simulink model "component_planner_adaptive_MPC"  (R2025a)
settings: Solver=FixedStepAuto  StartTime=0.0  StopTime=100  FixedStep=0.01  RelTol=1e-3  EnableMultiTasking=on
undefined symbols (not defined in the file): ego_target_velocity, MPC_prediction_horizon, tgt_traj_accel, tgt_traj_angle, tgt_traj_cte, tgt_traj_curv, tgt_traj_pos_x, tgt_traj_pos_y, tgt_traj_time, tgt_traj_velo, traj_valid_points
libraries: mpclib x1
settings Model: PauseTimes=61  NumberOfSteps=100  Creator=Z145442  LastModifiedBy=MarikL
settings SolverCC: AlgebraicLoopSolver=TrustRegion  PositivePriorityOrder=on  AutoInsertRateTranBlk=on
settings DataIOCC: SaveOutput=off  DSMLogging=off  SaveTime=off
settings OptimizationCC: EnhancedBackFolding=on  PassReuseOutputArgsAs=Individual arguments  ZeroExternalMemoryAtStartup=off  ZeroInternalMemoryAtStartup=off  MaxStackSize=2048  OptimizeBlockOrder=speed  DifferentSizesBufferReuse=on  OptimizationCustomize=off  EfficientTunableParamExpr=on
settings DebuggingCC: SignalInfNanChecking=error  MergeDetectMultiDrivingBlocksExec=none  ParameterOverflowMsg=none  ParameterTunabilityLossMsg=error  UnconnectedInputMsg=warning  UnconnectedOutputMsg=warning  UnconnectedLineMsg=warning  UniqueDataStoreMsg=warning  SFNoUnconditionalDefaultTransitionDiag=warning  ArithmeticOperatorsInVariantConditions=warning
settings HardwareCC: ProdBitPerPointer=32.0  ProdBitPerSizeT=32.0  ProdBitPerPtrDiffT=32.0  ProdLargestAtomicInteger=Long  ProdWordSize=32.0  ProdLongLongMode=on  ProdHWDeviceType=Infineon->TriCore
settings ModelReferenceCC: EnableRefExpFcnMdlSchedulingChecks=on  ModelReferenceNumInstancesAllowed=Single
settings SFSimCC: SimUseLocalCustomCode=off  MATLABDynamicMemAlloc=off  CustomCodeUndefinedFunction=UseInterfaceOnly
settings RTWCC: SystemTargetFile=ert.tlc  HardwareBoard=Infineon AURIX TC4x - TriBoards  GenCodeOnly=on  TemplateMakefile=ert_default_tmf  RTWUseLocalCustomCode=off  Toolchain=TASKING SmartCode for TriCore  GPUComputeCapability=3.5  Description=Embedded Coder
settings CodeAppCC: ForceParamTrailComments=on  IgnoreCustomStorageClasses=off  MaxIdLength=256.0  OperatorAnnotations=on  SimulinkDataObjDesc=on  SFDataObjDesc=on  InsertBlockDesc=on
settings ERTTargetCC: ExtModeTransport=0.0  ExtModeStaticAlloc=off  ExtModeMexFile=ext_comm  ExtModeIntrfLevel=Level1  InlinedParameterPlacement=Hierarchical  DynamicArrayContainerType=coder::array  SubcomponentCodeInterfacePackaging=Nonreusable function  SupportVariableSizeSignals=on

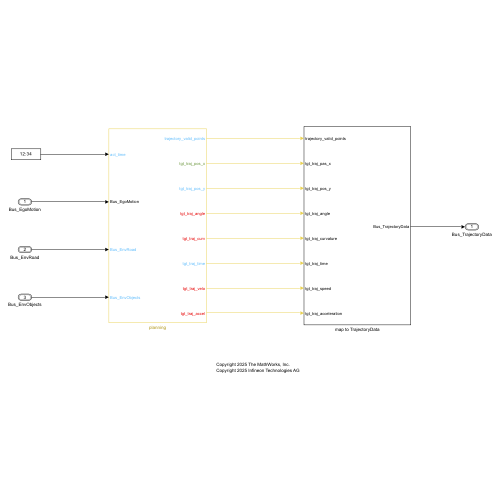
[thumbnail: Simulink's stored preview of the top-level diagram]
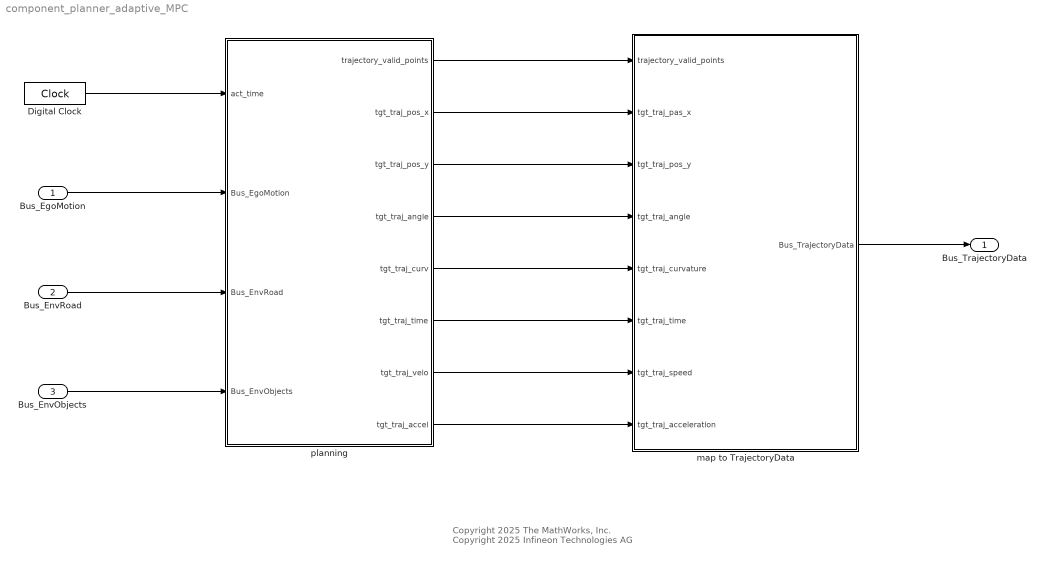
== system component_planner_adaptive_MPC ==
  note: Copyright 2025 The MathWorks, Inc.
      | Copyright 2025 Infineon Technologies AG
  Bus_EgoMotion : Inport  OutDataTypeStr=Bus: Bus_EgoMotion
  Bus_EnvRoad : Inport  Port=2  OutDataTypeStr=Bus: Bus_EnvRoad
  Bus_EnvObjects : Inport  Port=3  OutDataTypeStr=Bus: Bus_EnvObjects
  Digital Clock : DigitalClock  SampleTime=0.01
  map to TrajectoryData : Subsystem
  planning : Subsystem
  Bus_TrajectoryData : Outport  OutDataTypeStr=Bus: Bus_TrajectoryData  VectorParamsAs1DForOutWhenUnconnected=off
  wires:
  planning/6(tgt_traj_time) -> map to TrajectoryData/6(tgt_traj_time)
  planning/3(tgt_traj_pos_y) -> map to TrajectoryData/3(tgt_traj_pos_y)
  planning/5(tgt_traj_curv) -> map to TrajectoryData/5(tgt_traj_curvature)
  planning/8(tgt_traj_accel) -> map to TrajectoryData/8(tgt_traj_acceleration)
  planning/2(tgt_traj_pos_x) -> map to TrajectoryData/2(tgt_traj_pas_x)
  planning/4(tgt_traj_angle) -> map to TrajectoryData/4(tgt_traj_angle)
  planning/7(tgt_traj_velo) -> map to TrajectoryData/7(tgt_traj_speed)
  planning/1(trajectory_valid_points) -> map to TrajectoryData/1(trajectory_valid_points)
  map to TrajectoryData/1(Bus_TrajectoryData) -> Bus_TrajectoryData/1
  Digital Clock/1 -> planning/1(act_time)
  Bus_EnvRoad/1 -> planning/3(Bus_EnvRoad)
  Bus_EgoMotion/1 -> planning/2(Bus_EgoMotion)
  Bus_EnvObjects/1 -> planning/4(Bus_EnvObjects)

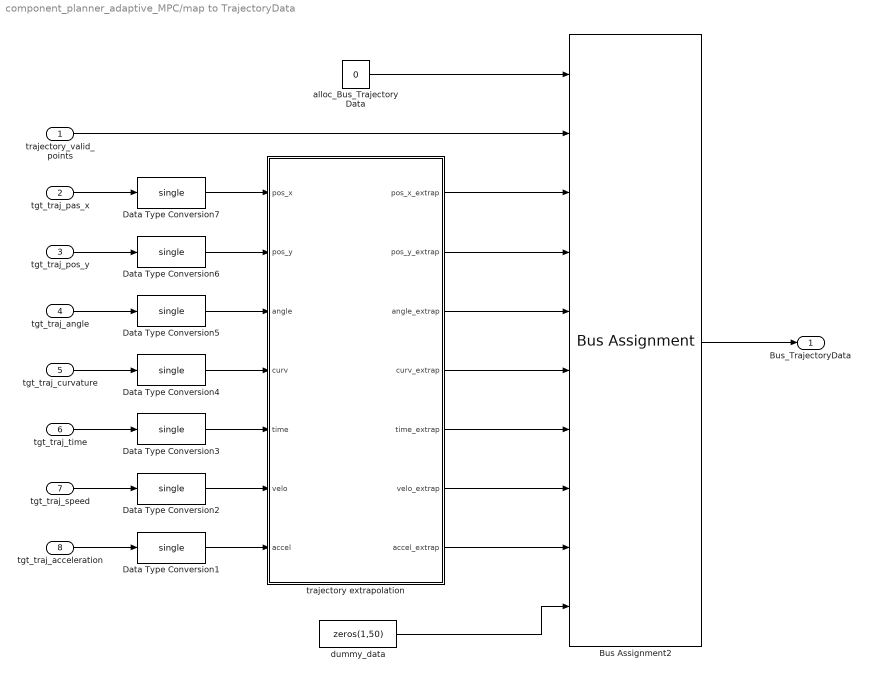
== system component_planner_adaptive_MPC/map to TrajectoryData ==
  trajectory_valid_points : Inport
  tgt_traj_pas_x : Inport  Port=2
  tgt_traj_pos_y : Inport  Port=3
  tgt_traj_angle : Inport  Port=4
  tgt_traj_curvature : Inport  Port=5
  tgt_traj_time : Inport  Port=6
  tgt_traj_speed : Inport  Port=7
  tgt_traj_acceleration : Inport  Port=8
  Bus Assignment2 : BusAssignment  AssignedSignals=traj_valid_points,tgt_traj_pos_x,tgt_traj_pos_y,tgt_traj_angle,tgt_traj_curv,tgt_traj_time,tgt_traj_velo,tgt_traj_accel,tgt_traj_cte
  Data Type Conversion{1..7} (7 alike) : DataTypeConversion  OutDataTypeStr=single  SaturateOnIntegerOverflow=off  RndMeth=Floor
  alloc_Bus_TrajectoryData : Constant  Value=0  OutDataTypeStr=Bus: Bus_TrajectoryData
  dummy_data : Constant  Value=zeros(1,50)  OutDataTypeStr=single
  trajectory extrapolation : MATLAB Function  TreatAsAtomicUnit=on  SystemSampleTime=0.01
  Bus_TrajectoryData : Outport  VectorParamsAs1DForOutWhenUnconnected=off
  wires:
  tgt_traj_curvature/1 -> Data Type Conversion4/1
  tgt_traj_angle/1 -> Data Type Conversion5/1
  tgt_traj_time/1 -> Data Type Conversion3/1
  tgt_traj_speed/1 -> Data Type Conversion2/1
  tgt_traj_acceleration/1 -> Data Type Conversion1/1
  tgt_traj_pos_y/1 -> Data Type Conversion6/1
  tgt_traj_pas_x/1 -> Data Type Conversion7/1
  trajectory_valid_points/1 -> Bus Assignment2/2
  trajectory extrapolation/5(time_extrap) -> Bus Assignment2/7
  trajectory extrapolation/4(curv_extrap) -> Bus Assignment2/6
  trajectory extrapolation/2(pos_y_extrap) -> Bus Assignment2/4
  Bus Assignment2/1 -> Bus_TrajectoryData/1
  alloc_Bus_TrajectoryData/1 -> Bus Assignment2/1
  trajectory extrapolation/6(velo_extrap) -> Bus Assignment2/8
  trajectory extrapolation/7(accel_extrap) -> Bus Assignment2/9
  trajectory extrapolation/3(angle_extrap) -> Bus Assignment2/5
  Data Type Conversion1/1 -> trajectory extrapolation/7(accel)
  Data Type Conversion2/1 -> trajectory extrapolation/6(velo)
  Data Type Conversion3/1 -> trajectory extrapolation/5(time)
  Data Type Conversion4/1 -> trajectory extrapolation/4(curv)
  Data Type Conversion5/1 -> trajectory extrapolation/3(angle)
  Data Type Conversion6/1 -> trajectory extrapolation/2(pos_y)
  Data Type Conversion7/1 -> trajectory extrapolation/1(pos_x)
  trajectory extrapolation/1(pos_x_extrap) -> Bus Assignment2/3
  dummy_data/1 -> Bus Assignment2/10

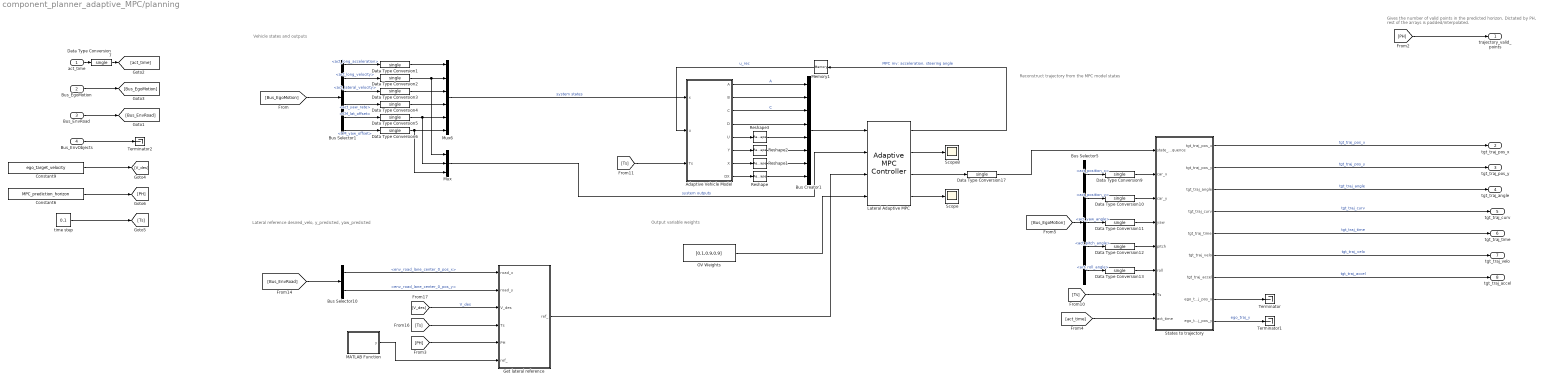
== system component_planner_adaptive_MPC/planning ==
  note: Output variable weights
  note: Reconstruct trajectory from the MPC model states
  note: Vehicle states and outputs
  note: Gives the number of valid points in the predicted horizon.
      | Dictated by PH, rest of the arrays is padded/interpolated.
  note: Lateral reference
      | desired_velo, y_predicted, yaw_predicted
  act_time : Inport
  Bus_EgoMotion : Inport  Port=2
  Bus_EnvRoad : Inport  Port=3
  Bus_EnvObjects : Inport  Port=4
  Adaptive Vehicle Model : MATLAB Function  TreatAsAtomicUnit=on  SystemSampleTime=0.1
  Bus Selector1 : BusSelector  OutputSignals=act_long_acceleration,act_long_velocity,act_lateral_velocity,act_yaw_rate,CM_lat_offset,CM_yaw_offset
  Bus Selector10 : BusSelector  OutputSignals=env_road_lane_center_0_pos_x,env_road_lane_center_0_pos_y
  Bus Selector5 : BusSelector  OutputSignals=act_position_x,act_position_y,act_yaw_angle,act_pitch_angle,act_roll_angle
  Bus Creator1 : BusCreator  Inputs=8  OutDataTypeStr=Bus: Bus_Model
      settings: InheritFromInputs=off
  Constant6 : Constant  Value=MPC_prediction_horizon  OutDataTypeStr=uint8
  Constant9 : Constant  Value=ego_target_velocity  OutDataTypeStr=single
  Data Type Conversion{1..7,9..13,17} (13 alike) : DataTypeConversion  OutDataTypeStr=single  SaturateOnIntegerOverflow=off  RndMeth=Floor
  Get lateral reference : MATLAB Function  TreatAsAtomicUnit=on  SystemSampleTime=0.1
  Lateral Adaptive MPC : mpclib/Adaptive MPC Controller  SCDEnableBlockLinearizationSpecification=on  mpcobj=mpc_latlon  enable_value=0  updateMPCinCallerWorkspace=on  md_inport=off  mv_inport=off  uref_inport=off  return_cost=on  return_mvseq=off  return_qpstatus=on  return_xseq=on  return_state=off  return_ovseq=off  state_inport=off  isltv_plant=off  umin_inport=off  umax_inport=off  ymin_inport=off  ymax_inport=off  cc_inport=off  ywt_inport=on  uwt_inport=off  duwt_inport=off  rhoeps_inport=off  pm_inport=off  MaximumP=10  HorizonChoice=FixedHorizon  BlockDataType=single  SampleTimeInherited=off  switch_inport=off
  MATLAB Function : MATLAB Function  TreatAsAtomicUnit=on
  Memory1 : Memory  InheritSampleTime=on
  Mux : Mux  Inputs=3
  Mux6 : Mux  Inputs=6
  OV Weights : Constant  Value=[0.1,0.9,0.9]  OutDataTypeStr=single
  Reshape{,1..3} (4 alike) : Reshape  OutputDimensionality=Column vector (2-D)
  Scope : Scope
      settings: ActiveDisplayYMinimum=0
  Scope8 : Scope
      settings: ActiveDisplayYMinimum=0
  States to trajectory : MATLAB Function  TreatAsAtomicUnit=on  SystemSampleTime=0.1
  Terminator : Terminator
  Terminator1 : Terminator
  Terminator2 : Terminator
  time step : Constant  Value=0.1  OutDataTypeStr=single
  trajectory_valid_points : Outport
  tgt_traj_pos_x : Outport  Port=2
  tgt_traj_pos_y : Outport  Port=3
  tgt_traj_angle : Outport  Port=4
  tgt_traj_curv : Outport  Port=5
  tgt_traj_time : Outport  Port=6
  tgt_traj_velo : Outport  Port=7
  tgt_traj_accel : Outport  Port=8
  wires:
  act_time/1 -> Data Type Conversion7/1
  Bus_EnvRoad/1 -> [Bus_EnvRoad]
  Bus_EgoMotion/1 -> [Bus_EgoMotion]
  Adaptive Vehicle Model/1(A) -> Bus Creator1/1  "A"
  Adaptive Vehicle Model/3(C) -> Bus Creator1/3  "C"
  Adaptive Vehicle Model/5(U) -> Reshape3/1
  Adaptive Vehicle Model/6(Y) -> Reshape2/1
  Adaptive Vehicle Model/7(X) -> Reshape1/1
  Adaptive Vehicle Model/8(DX) -> Reshape/1
  Bus Selector1/5 -> Data Type Conversion5/1  "<CM_lat_offset>"
  Mux6/1 -> Adaptive Vehicle Model/1(x)  "system states"
  Lateral Adaptive MPC/1 -> Memory1/1  "MPC mv: acceleration, steering angle"
  Bus Creator1/1 -> Lateral Adaptive MPC/1
  Mux/1 -> Lateral Adaptive MPC/2  "system outputs"
  Lateral Adaptive MPC/3 -> Data Type Conversion17/1
  Memory1/1 -> Adaptive Vehicle Model/2(u)  "u_rec"
  Reshape/1 -> Bus Creator1/8
  Reshape1/1 -> Bus Creator1/7
  Reshape2/1 -> Bus Creator1/6
  Reshape3/1 -> Bus Creator1/5
  [Bus_EgoMotion] -> Bus Selector5/1
  Bus Selector5/1 -> Data Type Conversion9/1  "<act_position_x>"
  Bus Selector5/2 -> Data Type Conversion10/1  "<act_position_y>"
  States to trajectory/1(tgt_traj_pos_x) -> tgt_traj_pos_x/1  "tgt_traj_pos_x"
  States to trajectory/2(tgt_traj_pos_y) -> tgt_traj_pos_y/1  "tgt_traj_pos_y"
  States to trajectory/3(tgt_traj_angle) -> tgt_traj_angle/1  "tgt_traj_angle"
  States to trajectory/4(tgt_traj_curv) -> tgt_traj_curv/1  "tgt_traj_curv"
  States to trajectory/5(tgt_traj_time) -> tgt_traj_time/1  "tgt_traj_time"
  States to trajectory/6(tgt_traj_velo) -> tgt_traj_velo/1  "tgt_traj_velo"
  States to trajectory/7(tgt_traj_accel) -> tgt_traj_accel/1  "tgt_traj_accel"
  Bus Selector5/3 -> Data Type Conversion11/1  "<act_yaw_angle>"
  Bus Selector5/4 -> Data Type Conversion12/1  "<act_pitch_angle>"
  Bus Selector5/5 -> Data Type Conversion13/1  "<act_roll_angle>"
  States to trajectory/8(ego_traj_pos_x) -> Terminator/1
  States to trajectory/9(ego_traj_pos_y) -> Terminator1/1  "ego_traj_y"
  Lateral Adaptive MPC/4 -> Scope/1
  Bus_EnvObjects/1 -> Terminator2/1
  Bus Selector10/2 -> Get lateral reference/2(road_y)  "<env_road_lane_center_0_pos_y>"
  [Bus_EnvRoad] -> Bus Selector10/1
  Bus Selector10/1 -> Get lateral reference/1(road_x)  "<env_road_lane_center_0_pos_x>"
  Adaptive Vehicle Model/4(D) -> Bus Creator1/4
  Adaptive Vehicle Model/2(B) -> Bus Creator1/2
  Bus Selector1/3 -> Data Type Conversion3/1  "<act_lateral_velocity>"
  Bus Selector1/4 -> Data Type Conversion4/1  "<act_yaw_rate>"
  [PH] -> Get lateral reference/5(PH)
  Bus Selector1/2 -> Data Type Conversion2/1  "<act_long_velocity>"
  Bus Selector1/1 -> Data Type Conversion1/1  "<act_long_acceleration>"
  [Bus_EgoMotion] -> Bus Selector1/1
  Bus Selector1/6 -> Data Type Conversion6/1  "<CM_yaw_offset>"
  Lateral Adaptive MPC/2 -> Scope8/1
  Constant6/1 -> [PH]
  [PH] -> trajectory_valid_points/1
  [V_des] -> Get lateral reference/3(V_des)  "V_des"
  Data Type Conversion1/1 -> Mux6/1
  Data Type Conversion2/1 -> Mux/1, Mux6/2
  Data Type Conversion3/1 -> Mux6/3
  Data Type Conversion4/1 -> Mux6/4
  Data Type Conversion5/1 -> Mux/2, Mux6/5
  Data Type Conversion6/1 -> Mux/3, Mux6/6
  OV Weights/1 -> Lateral Adaptive MPC/4
  [Ts] -> Adaptive Vehicle Model/3(Ts)
  Constant9/1 -> [V_des]
  time step/1 -> [Ts]
  [Ts] -> Get lateral reference/4(Ts)
  Get lateral reference/1(ref_) -> Lateral Adaptive MPC/3
  Data Type Conversion17/1 -> States to trajectory/1(state_sequence)
  [Ts] -> States to trajectory/7(Ts)
  [act_time] -> States to trajectory/8(act_time)
  MATLAB Function/1(y) -> Get lateral reference/6("ref_ ")
  Data Type Conversion9/1 -> States to trajectory/2(car_x)
  Data Type Conversion10/1 -> States to trajectory/3(car_y)
  Data Type Conversion11/1 -> States to trajectory/4(yaw)
  Data Type Conversion12/1 -> States to trajectory/5(pitch)
  Data Type Conversion13/1 -> States to trajectory/6(roll)
  Data Type Conversion7/1 -> [act_time]

== matlab function component_planner_adaptive_MPC/planning/States to trajectory ==
  data: state_sequence input; car_x input; tgt_traj_pos_x output; car_y input; yaw input; pitch input; roll input; tgt_traj_pos_y output; tgt_traj_angle output; tgt_traj_curv output; tgt_traj_time output; tgt_traj_velo output; tgt_traj_accel output; Ts input; act_time input; ego_traj_pos_x output; ego_traj_pos_y output
function [tgt_traj_pos_x, tgt_traj_pos_y, tgt_traj_angle, tgt_traj_curv, tgt_traj_time, tgt_traj_velo, tgt_traj_accel, ego_traj_pos_x, ego_traj_pos_y]  = fcn(state_sequence, car_x, car_y, yaw, pitch, roll, Ts, act_time)
%       - x: state vector
%           |lon_acc| - Longitudinal acceleration (ego)
%           |lon_velo| - Longitudinal velocity (ego)
%           |lat_velo| - Lateral velocity (ego)
%           |yaw_offset| - Yaw offset to the closest reference segment
%           |yaw_rate| - Yaw rate
%           |lat_offset| - Lateral offset to the closest reference segment

y_corr = state_sequence(1,6);
% remove the current state
state_sequence = state_sequence(2:end, :);
% state_sequence = state_sequence(1:end-1, :);

% TODO: return to dynamic (Simulink was complaining about the output size)
seq_len = 30; %size(state_sequence, 1);
t = linspace(0,(seq_len-1)*Ts,seq_len);

% integrate relative coordinates from velocity
lon_velo = state_sequence(:,2);
lon_velo(lon_velo < 1e-6) = 1e-6;
lat_velo = state_sequence(:,3);

sideslip = lat_velo./lon_velo;
sideslip(lon_velo < 5) = 0;
g = 9.8; % gravitational acceleration
n = 1; % vehicle's lateral load transfer coefficient (typically 0.5-1.5)
curv = sideslip ./ (lon_velo.^2 / g + sideslip * n);

x_ego = cumsum(lon_velo*Ts);
y_ego = state_sequence(:,5);% - y_corr; % cumsum(lat_velo*Ts); % 
% y_ego(1:3) = 0; % TODO: hotfix

[x_env, y_env] = transform_ego2env(x_ego, y_ego, car_x, car_y, yaw, pitch, roll);

% x_diff = diff([0; x_ego]);
% y_diff = diff([0; y_ego]);
x_diff = [diff(x_ego);0];
y_diff = [diff(y_ego);0];
% TODO: double-check the pos/neg direction
angle_ego = y_diff./x_diff; %atan(y_diff./x_diff);
angle_ego(x_diff < 0.0001) = 0;
% angle_ego(isnan(angle_ego)) = 0;
% angle_ego(~isfinite(angle_ego)) = 0;
angle_ego = atan(angle_ego);
% yaw_rate = state_sequence(:,4);
% angle_ego = cumsum(yaw_rate*Ts);
angle_env = angle_ego + yaw;


tgt_traj_pos_x = single(x_env);
tgt_traj_pos_y = single(y_env);
tgt_traj_angle = single(angle_env);
tgt_traj_curv = single(curv);
tgt_traj_time = single(act_time + t); % 0:Ts:(seq_len-1)*Ts;
tgt_traj_velo = single(lon_velo); %state_sequence(:,2);
tgt_traj_accel = single(state_sequence(:,1));
ego_traj_pos_x = single(x_ego);
ego_traj_pos_y = single(y_ego);

== matlab function component_planner_adaptive_MPC/planning/MATLAB Function ==
  data: y output
function y = fcn()
u = ones(30,3, 'single'); 
y = u;
end

== matlab function component_planner_adaptive_MPC/map to TrajectoryData/trajectory extrapolation ==
  settings: updateMethod=DISCRETE
  data: pos_x input; pos_y input; angle input; curv input; pos_x_extrap output; time input; pos_y_extrap output; velo input; accel input; angle_extrap output single; curv_extrap output; time_extrap output; velo_extrap output; accel_extrap output
function [pos_x_extrap, pos_y_extrap, angle_extrap, curv_extrap, time_extrap, velo_extrap, accel_extrap] = ...
    fcn(pos_x, pos_y, angle, curv, time, velo, accel)


[pos_x_extrap, pos_y_extrap, angle_extrap, curv_extrap, time_extrap, velo_extrap, accel_extrap] = ...
    extrapolate_trajectory(pos_x, pos_y, angle, curv, time, velo, accel);

== matlab function component_planner_adaptive_MPC/planning/Adaptive Vehicle Model ==
  data: x input; u input; A output; B output; C output; D output; U output; Y output; X output; DX output; Ts input
function [A,B,C,D,U,Y,X,DX] = fcn(x,u,Ts)

[A,B,C,D,U,Y,X,DX] = kinematic_system_single(x,u,Ts);

== matlab function component_planner_adaptive_MPC/planning/Get lateral reference ==
  data: ref_ output; road_x input; road_y input; V_des input; Ts input; PH input; ref_ input
function ref_ = fcn(road_x, road_y, V_des, Ts, PH, ref_)
ref_ = ref_;
temp = get_lateral_ref_single(road_x, road_y, V_des, Ts, PH); 
ref_ = temp;
